simulink model "sltestMaskedSubsystemExample"  (R2016a)
settings: Solver=ode23  StartTime=0.0  StopTime=80  MaxStep=0.01  RelTol=1e-3  AbsTol=1E-6
Description:
  | Bouncing Ball Model
  | 
  | This model calculates the trajectory, over time, of a ball thrown
  | upward with a velocity of 15 meters per second from a height of 10 m.
  | The model demonstrates the use of the 'ReinitDXDTwhenXreachesSaturation'
  | parameter in the Second-Order Integrator block to model this system.
  | This parameter, when set to 'on', forces a reinitialization of dx/dt
  | (velocity in the model) at the instant when x (position) reaches
  | saturation (i.e., when the ball hits the ground). The reinitialized value
  | is calculated by multiplying a coefficient of restitution times the ball
  | velocity, the instant before the ball hits the ground. The Memory block
  | in the calculation loop serves to capture the velocity of the ball just
  | before it hits the ground. The position of the ball is plotted in the
  | upper axis of the scope while the velocity of the ball is plotted in
  | the lower axis.
settings Model: Creator=The MathWorks, Inc.  LastModifiedBy=The MathWorks, Inc.
settings DataIOCC: MaxDataPoints=7500  SaveFormat=Array  SaveOutput=off  SignalLogging=off  DSMLogging=off  SaveTime=off
settings OptimizationCC: ExpressionDepthLimit=2147483647  EfficientFloat2IntCast=on
settings DebuggingCC: UnderspecifiedInitializationDetection=Classic  MergeDetectMultiDrivingBlocksExec=none  IgnoredZcDiagnostic=none  FcnCallInpInsideContextMsg=EnableAllAsWarning  StateNameClashWarn=warning
settings HardwareCC: ProdBitPerPointer=32  ProdLargestAtomicFloat=None  ProdIntDivRoundTo=Undefined  ProdEndianess=Unspecified  ProdWordSize=32  ProdHWDeviceType=32-bit Generic  TargetBitPerLong=64  TargetBitPerPointer=64  TargetLongLongMode=on  TargetIntDivRoundTo=Zero  TargetEndianess=LittleEndian  TargetWordSize=64  TargetHWDeviceType=MATLAB Host  ProdEqTarget=off
settings ModelReferenceCC: PropagateSignalLabelsOutOfModel=off
settings RTWCC: SystemTargetFile=rsim.tlc  TemplateMakefile=rsim_default_tmf  Description=Rapid Simulation Target
settings RSimTargetCC: ERTMultiwordTypeDef=System defined  ERTMultiwordLength=256
settings ConfigComp: CovModelRefEnable=Off

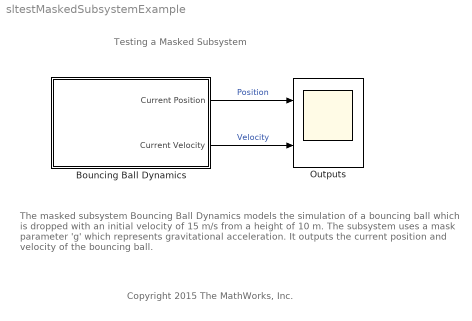
== system sltestMaskedSubsystemExample ==
  note: Testing a Masked Subsystem
  note: Copyright 2015 The MathWorks, Inc.
  note: The masked subsystem Bouncing Ball Dynamics models the simulation of a bouncing ball which is dropped with an initial velocity of 15 m/s from a height of 10 m. The subsystem uses a mask parameter 'g' which represents gravitational acceleration. It outputs the current position and velocity of the bouncing ball.
  Bouncing Ball Dynamics : Subsystem  mask{g=9.81}
      mask prompts: g "Gravitational Acceleration"
  Outputs : Scope  NumInputPorts=2
  wires:
  Bouncing Ball Dynamics/1(Current Position) -> Outputs/1  "Position"
  Bouncing Ball Dynamics/2(Current Velocity) -> Outputs/2  "Velocity"

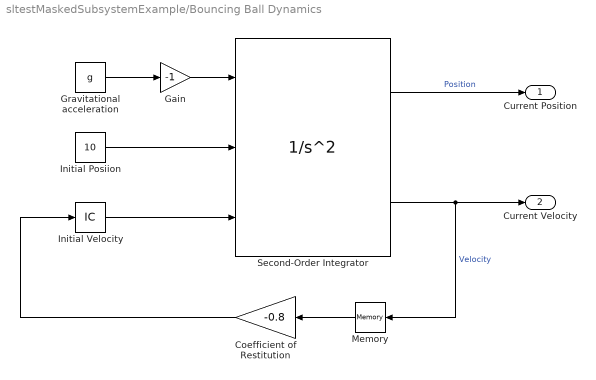
== system sltestMaskedSubsystemExample/Bouncing Ball Dynamics ==
  Coefficient of Restitution : Gain  Gain=-0.8
  Gain : Gain  Gain=-1
  Gravitational acceleration : Constant  Value=g  OutDataTypeStr=double
  "Initial Velocity " : InitialCondition  Value=15
  Initial Posiion : Constant  Value=10
  Memory : Memory
  Second-Order Integrator : SecondOrderIntegrator  ICSourceX=external  ICX=10.0  LimitX=on  LowerLimitX=0.0  StateNameX='Position'  ICSourceDXDT=external  StateNameDXDT='Velocity'  ReinitDXDTwhenXreachesSaturation=on
  Current Position : Outport
  Current Velocity : Outport  Port=2
  wires:
  Gravitational acceleration/1 -> Gain/1
  Coefficient of Restitution/1 -> "Initial Velocity "/1
  "Initial Velocity "/1 -> Second-Order Integrator/3
  Memory/1 -> Coefficient of Restitution/1
  Second-Order Integrator/2 -> Current Velocity/1, Memory/1  "Velocity"
  Second-Order Integrator/1 -> Current Position/1  "Position"
  Initial Posiion/1 -> Second-Order Integrator/2
  Gain/1 -> Second-Order Integrator/1
